simulink model "inclinaison_mag"  (R2021b)
settings: Solver=VariableStepAuto  StartTime=0.0  StopTime=10.0  RelTol=1e-3
undefined symbols (not defined in the file): WMM2010
libraries: aerolibgravity2 x1
settings Model: Creator=zayed  LastModifiedBy=zayed

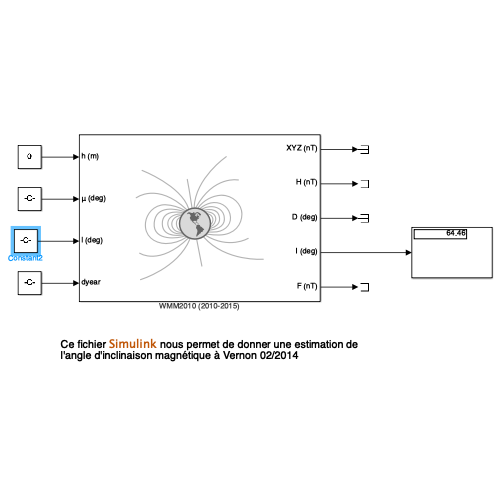
[thumbnail: Simulink's stored preview of the top-level diagram]
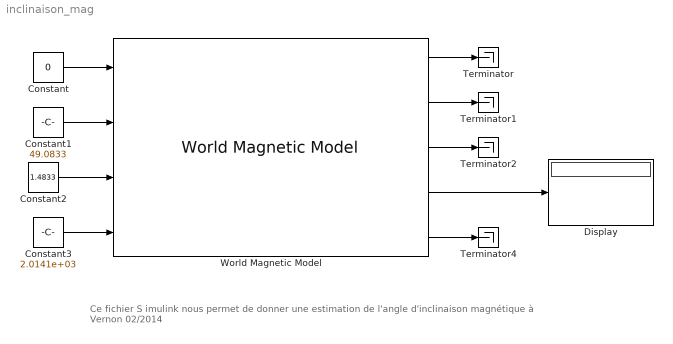
== system inclinaison_mag ==
  note: Ce fichier S imulink nous permet de donner une estimation de l'angle d'inclinaison magnétique à Vernon 02/2014
  Constant : Constant  Value=0  VectorParams1D=off
  Constant1 : Constant  Value=49.0833  VectorParams1D=off
  Constant2 : Constant  Value=1.4833  VectorParams1D=off
  Constant3 : Constant  Value=2.0141e+03  VectorParams1D=off
  Display : Display
  Terminator{,1..2,4} (4 alike) : Terminator
  World Magnetic Model : aerolibgravity2/World Magnetic Model  model=WMM2010 (2010-2015)  customFile='WMM2020.COF'  units=Metric (MKS)  time_in=on  month=January  day=1  year=2020  action=Error  h_out=on  dec_out=on  inc_out=on  ti_out=on
      settings: SourceProductBaseCode=AE
  wires:
  Constant/1 -> World Magnetic Model/1
  Constant1/1 -> World Magnetic Model/2
  Constant2/1 -> World Magnetic Model/3
  Constant3/1 -> World Magnetic Model/4
  World Magnetic Model/1 -> Terminator/1
  World Magnetic Model/2 -> Terminator1/1
  World Magnetic Model/3 -> Terminator2/1
  World Magnetic Model/4 -> Display/1
  World Magnetic Model/5 -> Terminator4/1
